simulink model "AssPosLaserPIMS_PIDck"  (R2020a)
settings: Solver=ode45  StartTime=0.0  StopTime=10  MaxStep=1e-4  RelTol=1e-3  EnableMultiTasking=on
values from neighbouring files (symbols this model uses):
  G0 = 40    [valeurs_assPosLaser.m]
  Kcapt = 447/G0    (= 11.175)    [valeurs_assPosLaser.m]
  Kp = 1    [valeurs_assPosLaser.m]
  Td = 1/wn    (= 0.00289372623803)    [valeurs_assPosLaser.m]
  Te = 1e-4    (= 0.0001)    [valeurs_assPosLaser.m]
  Ti = 1/wn    (= 0.00289372623803)    [valeurs_assPosLaser.m]
  wn = 2*pi*55    (= 345.575191895)    [valeurs_assPosLaser.m]
  xi = 0.8    [valeurs_assPosLaser.m]
libraries: simulink x3
settings Model: Creator=kulcsar  LastModifiedBy=Villou
settings DataIOCC: LimitDataPoints=on  SaveFormat=Array  ReturnWorkspaceOutputs=off
settings OptimizationCC: LifeSpan=inf
settings DebuggingCC: AlgebraicLoopMsg=none  UnderspecifiedInitializationDetection=Classic  MergeDetectMultiDrivingBlocksExec=none  SFUnexpectedBacktrackingDiag=warning  SFNoUnconditionalDefaultTransitionDiag=warning  SFExecutionAtInitializationDiag=none  ArithmeticOperatorsInVariantConditions=warning
settings HardwareCC: ProdBitPerPointer=32  ProdBitPerSizeT=32  ProdBitPerPtrDiffT=32  ProdLargestAtomicFloat=None  ProdIntDivRoundTo=Undefined  ProdEndianess=Unspecified  ProdWordSize=32  ProdHWDeviceType=32-bit Generic
settings ModelReferenceCC: PropagateSignalLabelsOutOfModel=off
settings SFSimCC: SimUseLocalCustomCode=off  CustomCodeUndefinedFunction=UseInterfaceOnly
settings RTWCC: RTWUseLocalCustomCode=off
settings CodeAppCC: StateflowObjectComments=on
settings GRTTargetCC: TargetLangStandard=C89/C90 (ANSI)
settings ConfigComp: CovMetricSettings=dw  CovHtmlReporting=on  CovSaveCumulativeToWorkspaceVar=on  CovSaveSingleToWorkspaceVar=on  CovExternalEMLEnable=off

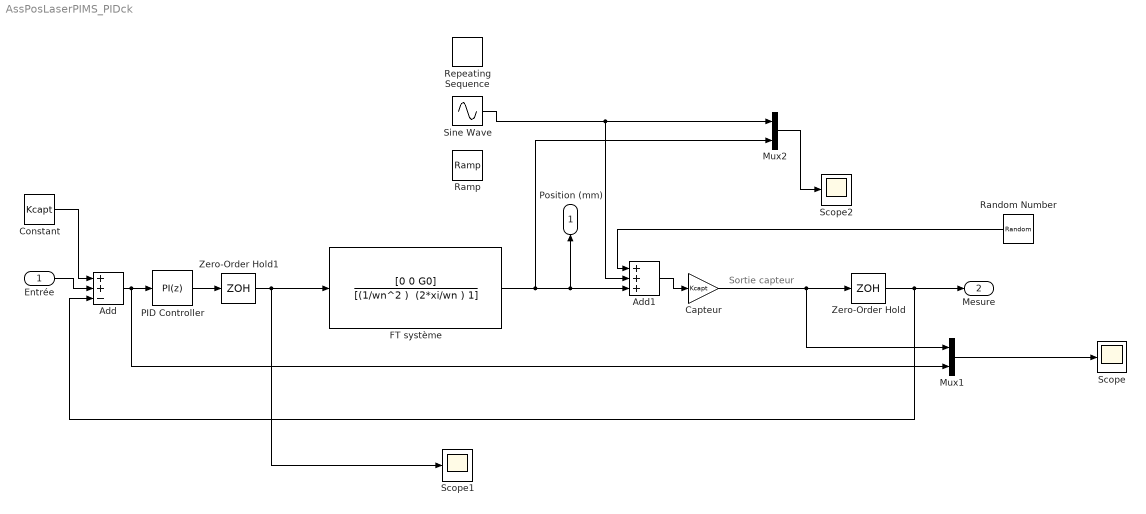
== system AssPosLaserPIMS_PIDck ==
  note: Sortie capteur
  Entrée : Inport
  Add : Sum  Inputs=++-
  Add1 : Sum  Inputs=+++
  Capteur : Gain  Gain=Kcapt
  Constant : Constant  Value=Kcapt
  "FT système " : TransferFcn  Numerator=[0 0 G0]  Denominator="[(1/wn^2 )  (2*xi/wn ) 1]"
  Mux1 : Mux  Inputs=2
  Mux2 : Mux  Inputs=2
  PID Controller : simulink/Continuous/PID Controller  Controller=PI  Form=Ideal  TimeDomain=Discrete-time  UseExternalTs=off  SampleTime=Te  IntegratorMethod=Backward Euler  FilterMethod=Trapezoidal  ControllerParametersSource=internal  P=Kp  I=1/Ti  D=Td  UseFilter=on  N=13426.8261863848  TunerSelectOption=Transfer Function Based (PID Tuner App)  InitialConditionSource=internal  InitialConditionForIntegrator=0  InitialConditionForFilter=0  DifferentiatorICPrevScaledInput=0  ExternalReset=none  TrackingMode=off  Kt=1  LimitOutput=off  UpperSaturationLimit=inf  LowerSaturationLimit=-inf  LinearizeAsGain=on  AntiWindupMode=none  Kb=1  POutMin=[]  POutMax=[]  IOutMin=[]  IOutMax=[]  DOutMin=[]  DOutMax=[]  NOutMin=[]  NOutMax=[]  SumOutMin=[]  SumOutMax=[]  SaturationOutMin=[]  SaturationOutMax=[]  PParamMin=[]  PParamMax=[]  IParamMin=[]  IParamMax=[]  DParamMin=[]  DParamMax=[]  NParamMin=[]  NParamMax=[]  KbParamMin=[]  KbParamMax=[]  KtParamMin=[]  KtParamMax=[]  KbOutMin=[]  KbOutMax=[]  KtOutMin=[]  KtOutMax=[]  IntegratorOutMin=[]  IntegratorOutMax=[]  FilterOutMin=[]  FilterOutMax=[]  SumI1OutMin=[]  SumI1OutMax=[]  SumI2OutMin=[]  SumI2OutMax=[]  SumI3OutMin=[]  SumI3OutMax=[]  SumI4OutMin=[]  SumI4OutMax=[]  SumDOutMin=[]  SumDOutMax=[]  DifferentiatorOutMin=[]  DifferentiatorOutMax=[]  FilterDiffOutCoefMin=[]  FilterDiffOutCoefMax=[]  ReciprocalOutMin=[]  ReciprocalOutMax=[]  SumDenOutMin=[]  SumDenOutMax=[]  SumNumOutMin=[]  SumNumOutMax=[]  DivideOutMin=[]  DivideOutMax=[]  UdiffTsProdOutMin=[]  UdiffTsProdOutMax=[]  NTsProdOutMin=[]  NTsProdOutMax=[]  UintegralTsProdOutMin=[]  UintegralTsProdOutMax=[]  UngainTsProdOutMin=[]  UngainTsProdOutMax=[]  IntegratorContinuousStateAttributes=''  IntegratorStateMustResolveToSignalObject=off  IntegratorRTWStateStorageClass=Auto  FilterContinuousStateAttributes=''  FilterStateMustResolveToSignalObject=off  FilterRTWStateStorageClass=Auto  ParallelPVariant=Passthrough  IdealPVariant=InternalParameters  IVariant=InternalParameters  DVariant=Disabled  IntegratorVariant=Discrete  SatVariant=Disabled  AWVariant=Passthrough  PCopyVariant=Disabled  TRVariant=Disabled  FdbkBlocksVariant=Forward  IdealPFdbkVariant=Disabled  SatFdbkVariant=Disabled  DerivativeFilterVariant=Disabled  NVariant=Disabled  NCopyVariant=Disabled_SignalSpec  FilterICVariant=Disabled  IntegratorICVariant=InternalICs  ExternalResetVariant=Disabled  TRSumVariant=Passthrough  SumFdbkVariant=Disabled  SumVariant=Sum_PI  TsampFilterVariant=InternalTs  TsampNgainVariant=Passthrough  TsampIntegralVariant=Passthrough
  Ramp : simulink/Sources/Ramp  slope=1  start=0  InitialOutput=0
  Random Number : RandomNumber  Variance=0.01/Kcapt  SampleTime=Te
  Repeating Sequence : simulink/Sources/Repeating Sequence  rep_seq_t=[0:Te:1000*Te]  rep_seq_y=[0:Te:499*Te, 499*Te:-Te:-Te]*1000
  Scope : Scope
  Scope1 : Scope
  Scope2 : Scope
  Sine Wave : Sin  Amplitude=0.5  Frequency=2*pi*2  SampleTime=0
  Zero-Order Hold : ZeroOrderHold  SampleTime=Te
  Zero-Order Hold1 : ZeroOrderHold  SampleTime=Te
  Position (mm) : Outport  VectorParamsAs1DForOutWhenUnconnected=off
  Mesure : Outport  Port=2  VectorParamsAs1DForOutWhenUnconnected=off
  wires:
  Entrée/1 -> Add/2
  "FT système "/1 -> Mux2/2, Add1/3, Position (mm)/1
  Add/1 -> Mux1/2, PID Controller/1
  Constant/1 -> Add/1
  Mux1/1 -> Scope/1
  PID Controller/1 -> Zero-Order Hold1/1
  Zero-Order Hold1/1 -> "FT système "/1, Scope1/1
  Add1/1 -> Capteur/1
  Zero-Order Hold/1 -> Add/3, Mesure/1
  Mux2/1 -> Scope2/1
  Random Number/1 -> Add1/1
  Sine Wave/1 -> Add1/2, Mux2/1
  Capteur/1 -> Mux1/1, Zero-Order Hold/1
